simulink model "Sim"  (R2021a)
settings: Solver=VariableStepAuto  StartTime=0.0  StopTime=time  RelTol=1e-3
values from neighbouring files (symbols this model uses):
  dt = 0.005    [Identify.m]
  theta = inv(phi_M'*phi_M)*phi_M'*ip'    [Identify.m]
libraries: simulink x1
settings Model: Creator=1  LastModifiedBy=1

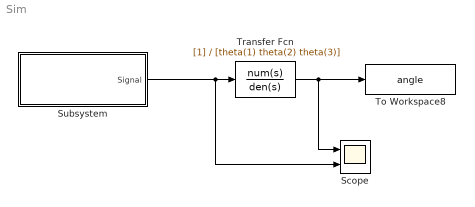
== system Sim ==
  Scope : Scope  NumInputPorts=2
  Subsystem : Subsystem  mask{st=dt, amp=0.6, freq=1}
      mask prompts: st "Sample time(s)"; amp "Amplitude"; freq "Frequency(Hz)"
      mask help: Sample time：必须和系统周期保持一致
      mask Display: disp('自定义方波信号')
  To Workspace8 : ToWorkspace  VariableName=angle  SampleTime=0.005
  Transfer Fcn : TransferFcn  Denominator=[theta(1) theta(2) theta(3)]
  wires:
  Transfer Fcn/1 -> To Workspace8/1, Scope/1
  Subsystem/1(Signal) -> Scope/2, Transfer Fcn/1

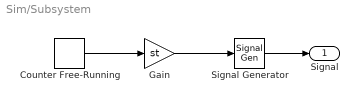
== system Sim/Subsystem ==
  Counter Free-Running : simulink/Sources/Counter Free-Running  NumBits=32  tsamp=-1
  Gain : Gain  Gain=st  OutDataTypeStr=double
  Signal Generator : SignalGenerator  WaveForm=square  TimeSource=Use external signal  Amplitude=amp  Frequency=freq
  Signal : Outport
  wires:
  Counter Free-Running/1 -> Gain/1
  Signal Generator/1 -> Signal/1
  Gain/1 -> Signal Generator/1
